simulink model "parallel_SST_model"  (R2024b)
settings: Solver=FixedStepAuto  StartTime=0.0  StopTime=150000  FixedStep=60  RelTol=1e-3
settings Model: VariantFading=off  Creator=mouzounb  LastModifiedBy=nerotb
settings OptimizationCC: StrengthReduction=on  PassReuseOutputArgsAs=Individual arguments  OptimizeBlockOrder=speed  OptimizationPriority=Speed  OptimizationCustomize=off  MultiThreadedLoops=on  AutoScheduleForLoops=on  EfficientTunableParamExpr=on
settings DebuggingCC: ParameterTunabilityLossMsg=error
settings RTWCC: Description=Embedded Coder  SystemTargetFile=ert.tlc  GenCodeOnly=on  TemplateMakefile=ert_default_tmf  BuildConfiguration=Faster Runs  CodeProfilingInstrumentation=coarse
settings CodeAppCC: ForceParamTrailComments=on  IgnoreCustomStorageClasses=off  OperatorAnnotations=on  SimulinkDataObjDesc=on  SFDataObjDesc=on  ParamNamingRule=UpperCase  InsertBlockDesc=on  BlockCommentType=BlockSIDComment  MATLABSourceComments=on
settings ERTTargetCC: TargetLangStandard=C99 (ISO)  GenerateSampleERTMain=on  SupportContinuousTime=on  SupportVariableSizeSignals=on  InlinedParameterPlacement=Hierarchical  ERTCustomFileTemplate=example_file_process.tlc  RateTransitionBlockCode=Function  IndentStyle=Allman

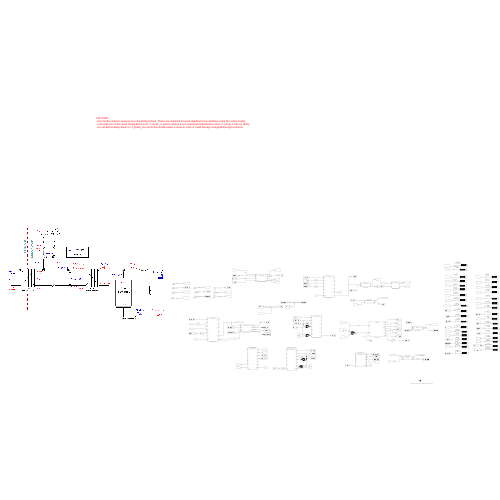
[thumbnail: Simulink's stored preview of the top-level diagram]
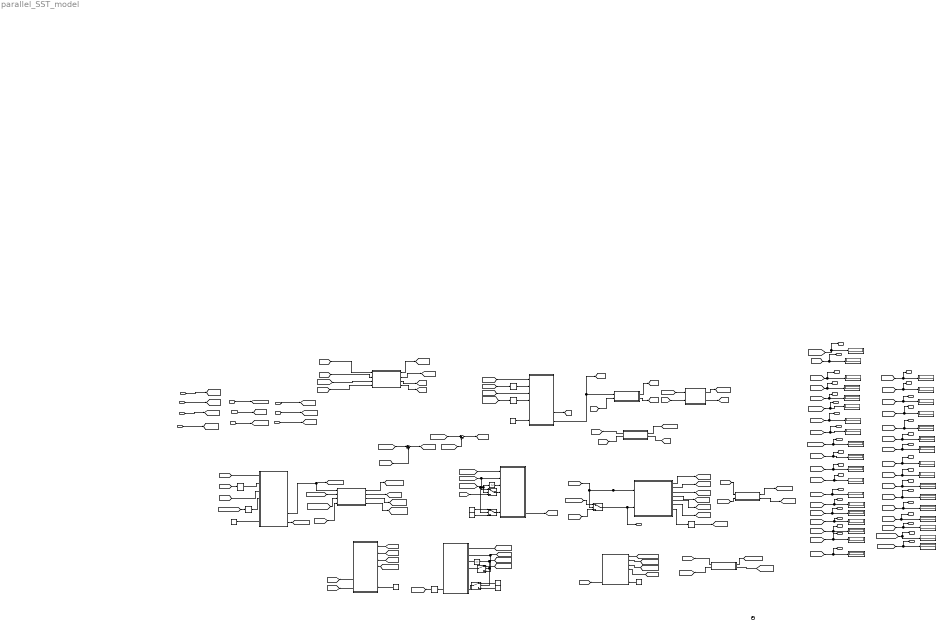
== system parallel_SST_model ==
  note: This clock is needed at the Python interface creation step, just keep it
  note: CAUTION:
      | - this model contains several one step Delay blocks. These are required to break algebraic loop and thus solve the entire model.
      | - note that one of the used Delay block is for T_stock_n, which creates a non symmetrical behaviour since T_stock_1 has no delay
      | - do not define delay block on T_DHW_out since this would cause a mess in case of rapid storage charge/discharge inversion
  m_prim : Inport  OutMin=0
  T_prim_in : Inport  Port=2
  m_SH_dir : Inport  Port=3  OutMin=0
  m_SH_3V : Inport  Port=4  OutMin=0
  m_DHW_sec : Inport  Port=5  OutMin=0
  m_DHW_w : Inport  Port=6  OutMin=0
  m_DHW_recirc : Inport  Port=7  OutMin=0  Interpolate=off
  T_cold : Inport  Port=8
  m_DHW_dir : Inport  Port=9  OutMin=0
  m_DHW_3V : Inport  Port=10  OutMin=0
  Abs : Abs  SaturateOnIntegerOverflow=off
  Abs1 : Abs  SaturateOnIntegerOverflow=off
  Clock : Clock
  Constant : Constant  Value=0
  Constant{1..4,6..7} (6 alike) : Constant
  Constant5 : Constant  Value=0
  DHW by-pass valve : Subsystem  ReferencedSubsystem=three_way_valve  unknown_m=m_3  unknown_T=T_3
  DHW cold water refill : Subsystem  ReferencedSubsystem=three_way_valve  unknown_m=m_3  unknown_T=T_3
  DHW heat exchanger : Subsystem  ReferencedSubsystem=heat_exchanger  U=1000  A=100
  DHW return pipe : Subsystem  ReferencedSubsystem=thermal_pipe  m_min=0.1  insulation_class=4  D=0.03  L=50  T_duct=15
  DHW storage : Subsystem  ReferencedSubsystem=storage_TC  D=1  H=1.5  n=61  V_var=60  V_min=10  U=5  eps=2  T_amb=20
  DHW storage bottom valve : Subsystem  ReferencedSubsystem=three_way_valve  unknown_m=m_3  unknown_T=T_3
  DHW storage top valve : Subsystem  ReferencedSubsystem=three_way_valve  unknown_m=m_3  unknown_T=T_3
  DHW supply pipe : Subsystem  ReferencedSubsystem=thermal_pipe  m_min=0.1  insulation_class=4  D=0.03  L=50  T_duct=15
  Delay{,1..2,5..7} (6 alike) : Delay  DelayLength=1  InputProcessing=Columns as channels (frame based)
  Display{1..3,12..17,19..38,76..81} (35 alike) : Display
  Primary heat exchanger : Subsystem  ReferencedSubsystem=heat_exchanger  U=1000  A=100
  SH by-pass valve : Subsystem  ReferencedSubsystem=three_way_valve  unknown_m=m_3  unknown_T=T_3
  SH return pipe : Subsystem  ReferencedSubsystem=thermal_pipe  m_min=0.09  insulation_class=4  D=0.05  L=50  T_duct=15
  SH supply pipe : Subsystem  ReferencedSubsystem=thermal_pipe  m_min=0.09  insulation_class=4  D=0.05  L=50  T_duct=15
  SH thermal emitters : Subsystem  ReferencedSubsystem=thermal_emitters  m_min=0.09  n_radiators=12  n_tubes=136  D=0.02  L=0.46  U=10  T_air=20
  SH-DHW return valve : Subsystem  ReferencedSubsystem=three_way_valve  unknown_m=m_3  unknown_T=T_3
  Sum : Sum  Inputs=|++
  Sum1 : Sum  Inputs=|+-
  Switch{,1..4} (5 alike) : Switch  Criteria=u2 > Threshold  SaturateOnIntegerOverflow=off  InputSameDT=off
  T_sec_in : Outport
  T_DHW_out : Outport  Port=2
  T_out : Outport  Port=3
  T_DHW_sec_out : Outport  Port=4
  T_DHW_sec_in : Outport  Port=5
  T_DHW_prim_in : Outport  Port=6
  T_DHW_prim_out : Outport  Port=7
  T_SH_out : Outport  Port=8
  T_SH_in : Outport  Port=9
  T_prim_out : Outport  Port=10
  T_sec_out : Outport  Port=11
  T_SH_emitter_out : Outport  Port=12
  T_stor_n : Outport  Port=13
  Q_SH : Outport  Port=14
  Q_primary_HX : Outport  Port=15
  Q_DHW_HX : Outport  Port=16
  m_DHW : Outport  Port=17
  Q_SH_supply : Outport  Port=18
  Q_SH_return : Outport  Port=19
  T_stor_out : Outport  Port=20
  T_stor_avg : Outport  Port=21
  T_stor_mid : Outport  Port=22
  T_stor_std : Outport  Port=23
  T_stor_half : Outport  Port=24
  T_stor_1 : Outport  Port=25
  m_DHW_prim : Outport  Port=26
  m_sec : Outport  Port=27
  m_SH : Outport  Port=28
  Q_DHW_supply : Outport  Port=29
  Q_DHW_return : Outport  Port=30
  efficiency_primary_HX : Outport  Port=31
  efficiency_DHW_HX : Outport  Port=32
  T_DHW_in : Outport  Port=33
  T_SH_emitter_in : Outport  Port=34
  T_stor_in : Outport  Port=35
  m_DHW_stor : Outport  Port=36
  wires:
  DHW storage/4 -> [T_stor_std]
  [T_prim_in] -> Primary heat exchanger/3  "T_prim_in"
  SH thermal emitters/1 -> [T_SH_emitter_out]  "T_out_emet"
  DHW storage/5 -> [T_stor_half]
  DHW supply pipe/1 -> [T_out_DHW_supply]  "T_in_DHW"
  [m_DHW] -> DHW supply pipe/2  "m_DHW"
  DHW heat exchanger/4 -> [efficiency_DHW_HX]  "efficiency_primary_HX"
  Primary heat exchanger/3 -> [Q_primary_HX]
  [m_prim] -> Primary heat exchanger/1  "m_prim"
  DHW storage/2 -> [T_stor_avg]
  [T_DHW_in] -> DHW supply pipe/1
  DHW storage/3 -> [T_stor_mid]
  [m_DHW_w] -> DHW cold water refill/3
  DHW heat exchanger/3 -> [Q_DHW_HX]  "Q_primary_HX"
  [m_DHW_sec] -> DHW heat exchanger/2
  [T_sec_in] -> Primary heat exchanger/4
  Primary heat exchanger/2 -> [T_sec_out]  "T_sec_out"
  [m_SH] -> SH thermal emitters/2  "m_SH"
  DHW heat exchanger/1 -> [T_DHW_prim_out]  "T_1_out"
  [T_cold] -> DHW cold water refill/4
  SH thermal emitters/2 -> [Q_SH]  "Q"
  [T_DHW_out] -> DHW cold water refill/2
  [T_DHW_prim_in] -> DHW heat exchanger/3
  DHW return pipe/1 -> [T_DHW_out]  "T_out_DHW"
  Primary heat exchanger/4 -> [efficiency_primary_HX]  "efficiency_primary_HX"
  [T_out_DHW_supply] -> DHW return pipe/1
  DHW heat exchanger/2 -> [T_DHW_sec_out]  "T_DHW_sec_out"
  DHW storage/1 -> [T_stor_out]
  [m_DHW_recirc] -> DHW return pipe/2  "m_DHW_recirc"
  Primary heat exchanger/1 -> [T_prim_out]  "T_prim_out"
  [T_SH_emitter_in] -> SH thermal emitters/1
  [T_out] -> Switch/3
  Switch/1 -> DHW storage/2, T_stor_in/1  "T_stock_in"
  m_prim/1 -> [m_prim]  "m_prim"
  m_DHW_dir/1 -> [m_DHW_dir]  "m_DHW_dir"
  T_cold/1 -> [T_cold]  "T_cold"
  m_DHW_w/1 -> [m_DHW_w]  "m_DHW_w"
  m_DHW_3V/1 -> [m_DHW_3V]  "m_DHW_3V"
  m_SH_3V/1 -> [m_SH_3V]  "m_SH_3V"
  m_SH_dir/1 -> [m_SH_dir]  "m_SH_dir"
  [T_SH_in] -> T_SH_in/1, Display81/1
  [T_stor_std] -> T_stor_std/1, Display26/1
  [Q_DHW_return] -> Q_DHW_return/1, Display34/1
  [Q_SH_supply] -> Q_SH_supply/1, Display21/1
  [T_stor_n] -> T_stor_n/1, Display14/1
  [efficiency_DHW_HX] -> efficiency_DHW_HX/1, Display37/1
  [T_stor_half] -> T_stor_half/1, Display27/1
  [T_sec_in] -> Display35/1, T_sec_in/1
  [m_DHW] -> m_DHW/1, Display19/1
  [T_DHW_out] -> T_DHW_out/1, Display20/1
  [Q_DHW_supply] -> Q_DHW_supply/1, Display33/1
  [T_out] -> T_out/1, Display31/1
  [T_stor_mid] -> T_stor_mid/1, Display25/1
  [m_sec] -> m_sec/1, Display30/1
  [Q_primary_HX] -> Q_primary_HX/1, Display16/1
  [efficiency_primary_HX] -> Display36/1, efficiency_primary_HX/1
  [T_stor_avg] -> T_stor_avg/1, Display24/1
  [T_DHW_sec_in] -> T_DHW_sec_in/1, Display77/1
  [T_sec_out] -> T_sec_out/1, Display13/1
  [T_SH_out] -> T_SH_out/1, Display80/1
  [T_DHW_prim_in] -> T_DHW_prim_in/1, Display78/1
  [m_SH] -> m_SH/1, Display32/1
  [T_prim_out] -> T_prim_out/1, Display12/1
  [Q_SH] -> Q_SH/1, Display15/1
  [Q_SH_return] -> Q_SH_return/1, Display22/1
  [T_stor_1] -> T_stor_1/1, Display28/1
  [T_DHW_sec_out] -> T_DHW_sec_out/1, Display76/1
  [Q_DHW_HX] -> Q_DHW_HX/1, Display17/1
  [T_SH_emitter_out] -> T_SH_emitter_out/1, Display38/1
  [T_stor_out] -> T_stor_out/1, Display23/1
  [T_DHW_prim_out] -> T_DHW_prim_out/1, Display79/1
  [m_DHW_prim] -> m_DHW_prim/1, Display29/1
  [m_DHW_recirc] -> DHW cold water refill/1
  DHW return pipe/2 -> [Q_DHW_return]
  DHW supply pipe/2 -> [Q_DHW_supply]
  SH supply pipe/1 -> [T_SH_emitter_in]
  [T_SH_emitter_out] -> SH return pipe/1
  [m_SH] -> SH return pipe/2  "m_SH"
  SH return pipe/1 -> [T_SH_out]
  [m_SH] -> SH supply pipe/2  "m_SH"
  [T_DHW_sec_out] -> Switch/1
  [T_DHW_in] -> T_DHW_in/1, Display1/1
  [T_SH_emitter_in] -> Display3/1, T_SH_emitter_in/1
  SH return pipe/2 -> [Q_SH_return]
  SH supply pipe/2 -> [Q_SH_supply]
  [m_sec] -> Primary heat exchanger/2  "m_prim"
  [m_DHW_recirc] -> Sum/1  "m_DHW_recirc"
  [m_DHW_w] -> Sum/2
  T_prim_in/1 -> [T_prim_in]  "T_prim_in"
  [m_DHW_sec] -> Sum1/1  "m_DHW_sec"
  Sum/1 -> [m_DHW]  "m_DHW"
  SH by-pass valve/5 -> [m_SH]  "m_3"
  [T_sec_out] -> Delay2/1
  Constant2/1 -> SH by-pass valve/7
  SH by-pass valve/6 -> [T_SH_in], SH supply pipe/1  "T_3"
  [m_SH_3V] -> SH by-pass valve/3
  [T_sec_out] -> Delay/1
  [T_DHW_prim_out] -> Delay1/1
  Constant1/1 -> DHW by-pass valve/7
  DHW by-pass valve/6 -> [T_DHW_prim_in]  "T_3"
  DHW by-pass valve/5 -> [m_DHW_prim], DHW heat exchanger/1  "m_3"
  [m_SH_dir] -> SH-DHW return valve/1
  [m_DHW_dir] -> SH-DHW return valve/3
  [T_DHW_prim_out] -> SH-DHW return valve/4
  Constant3/1 -> SH-DHW return valve/7
  SH-DHW return valve/6 -> [T_sec_in]  "T_3"
  SH-DHW return valve/5 -> [m_sec]  "m_3"
  [m_DHW] -> DHW storage bottom valve/1
  [T_out] -> DHW storage bottom valve/2, Switch4/3
  Switch1/1 -> DHW storage bottom valve/7
  Constant/1 -> Switch1/3
  Constant4/1 -> Switch1/1
  DHW storage bottom valve/6 -> Delay6/1  "T_3"
  [m_DHW_sec] -> DHW storage top valve/1
  Switch2/1 -> DHW storage top valve/7
  Constant5/1 -> Switch2/1
  Constant6/1 -> Switch2/3
  DHW storage top valve/6 -> [T_DHW_in]  "T_3"
  DHW storage/7 -> Delay5/1
  [T_DHW_sec_in] -> DHW heat exchanger/4
  [T_SH_out] -> Delay7/1
  m_DHW_sec/1 -> [m_DHW_sec]  "m_DHW_sec"
  [T_DHW_sec_out] -> Switch3/1, DHW storage top valve/2
  [m_DHW_stor] -> Abs/1, Switch3/2, Switch2/2
  [T_stor_n] -> Switch3/3
  Switch3/1 -> DHW storage top valve/4
  [m_DHW_stor] -> Switch1/2, Switch4/2, Abs1/1
  [T_stor_1] -> Switch4/1
  Switch4/1 -> DHW storage bottom valve/4
  DHW cold water refill/6 -> [T_out]
  [m_DHW_stor] -> Switch/2, DHW storage/1
  DHW storage/6 -> [T_stor_1]
  Delay5/1 -> [T_stor_n]
  Delay6/1 -> [T_DHW_sec_in]
  [T_SH_out] -> SH-DHW return valve/2
  Delay2/1 -> SH by-pass valve/2
  [m_SH_dir] -> SH by-pass valve/1
  Delay7/1 -> SH by-pass valve/4
  [m_DHW_dir] -> DHW by-pass valve/1
  [m_DHW_3V] -> DHW by-pass valve/3
  Delay/1 -> DHW by-pass valve/2
  Delay1/1 -> DHW by-pass valve/4
  Abs/1 -> DHW storage top valve/3
  Abs1/1 -> DHW storage bottom valve/3
  m_DHW_recirc/1 -> [m_DHW_recirc]  "m_DHW_recirc"
  Sum1/1 -> [m_DHW_stor]  "m_DHW_stor"
  [m_DHW] -> Sum1/2
  [m_DHW_stor] -> m_DHW_stor/1, Display2/1
  Constant7/1 -> DHW cold water refill/7
